simulink model "me132Hw1Q5_BallTrajectoryDrag"  (R2021a)
settings: Solver=VariableStepAuto  StartTime=0.0  StopTime=10.0  RelTol=1e-3
values from neighbouring files (symbols this model uses):
  g = -9.81    [hw1Q4.m]    (also in hw1Q5.m)
  mass = 0.3    [hw1Q4.m]    (also in hw1Q5.m)
  v0_x = 35 * cosd(65)    [hw1Q4.m]    (also in hw1Q5.m)
  v0_y = 35 * sind(65)    [hw1Q4.m]    (also in hw1Q5.m)
settings Model: Creator=kaiyu  LastModifiedBy=kaiyu

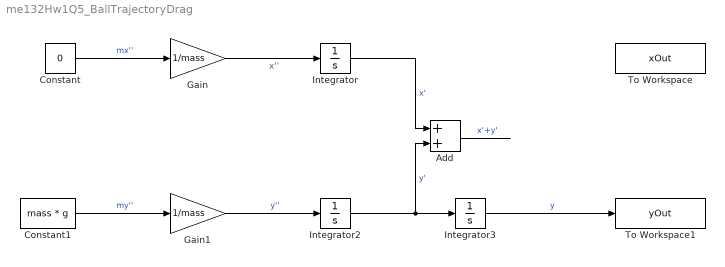
== system me132Hw1Q5_BallTrajectoryDrag ==
  note: x''
  Add : Sum
  Constant : Constant  Value=0
  Constant1 : Constant  Value=mass * g
  Gain : Gain  Gain=1/mass
  Gain1 : Gain  Gain=1/mass
  Integrator : Integrator  InitialCondition=v0_x
  Integrator2 : Integrator  InitialCondition=v0_y
  Integrator3 : Integrator
  To Workspace : ToWorkspace  VariableName=xOut  SaveFormat=Timeseries  SampleTime=-1
  To Workspace1 : ToWorkspace  VariableName=yOut  SaveFormat=Timeseries  SampleTime=-1
  wires:
  Constant1/1 -> Gain1/1  "my''"
  Constant/1 -> Gain/1  "mx''"
  Gain1/1 -> Integrator2/1  "y''"
  Integrator/1 -> Add/1  "x'"
  Integrator3/1 -> To Workspace1/1  "y"
  Integrator2/1 -> Add/2, Integrator3/1  "y'"
  Gain/1 -> Integrator/1
  Add/1 -> ?  "x'+y'"
